simulink model "Homework1_Sistem_mar"  (R2017b)
settings: Solver=VariableStepAuto  StartTime=0.0  StopTime=300.0  RelTol=1e-3
settings Model: Creator=Juan Salguero  LastModifiedBy=El Rubio
settings CodeAppCC: StateflowObjectComments=on

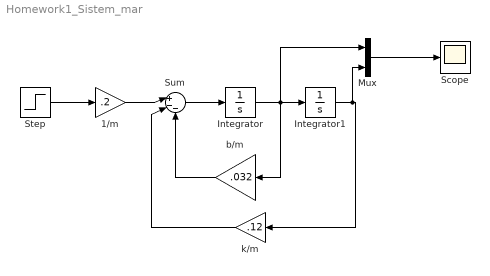
== system Homework1_Sistem_mar ==
  1/m : Gain  Gain=.2
  Integrator : Integrator
  Integrator1 : Integrator
  Mux : Mux  Inputs=2
  Scope : Scope
  Step : Step  Time=5  Before=50  After=0  SampleTime=0
  Sum : Sum  Inputs=|+--
  b/m : Gain  Gain=.032
  k/m : Gain  Gain=.12
  wires:
  Step/1 -> 1/m/1
  1/m/1 -> Sum/1
  Sum/1 -> Integrator/1
  Integrator/1 -> Mux/1, b/m/1, Integrator1/1
  b/m/1 -> Sum/3
  Integrator1/1 -> Mux/2, k/m/1
  k/m/1 -> Sum/2
  Mux/1 -> Scope/1
